simulink model "motor_1"  (R2023a)
settings: Solver=ode15s  StartTime=0.0  StopTime=sim_end_time  MaxStep=.0001  RelTol=1e-3
values from neighbouring files (symbols this model uses):
  alpha_cu = 3.9 *10^-3    (= 0.0039)    [BLDC_Motor_params_03.m]    (also in DC_Motor_params_01.m; DC_Motor_params_02.m; DC_Motor_params_04.m; DC_Motor_params_05.m)
  b_m1 = .01    (= 0.01)    [DC_Motor_params_01.m]
  C_t1 = 19.57    [DC_Motor_params_01.m]
  ENABLE_SATURATIONS = 1    [run_flags.m]
  J_eq1 = J_1 + 1/8 * m_1 * d_1^2 / r_1^2    [DC_Motor_params_01.m]
  K_d1 = 0.022261    [PID_tuning.m]
  k_e1 = 0.25    [DC_Motor_params_01.m]
  K_i1 = 0    [PID_tuning.m]
  K_p1 = 6.6674    [PID_tuning.m]
  k_t1 = 0.25    [DC_Motor_params_01.m]
  L_a1 = 7.5*10^-3    (= 0.0075)    [DC_Motor_params_01.m]
  r_1 = 25    [DC_Motor_params_01.m]
  r_a1_20 = 0.5    [DC_Motor_params_01.m]
  res_term_1 = 9.58    [DC_Motor_params_01.m]
  T_s0_1 = 20    [use_machine_1.m]    (also in use_solo_motor_1.m)
  theta_m0_1 = 0    [use_machine_1.m]    (also in use_solo_motor_1.m)
  voltage_1 = 12    [DC_Motor_params_01.m]
settings Model: Creator=Usuario  LastModifiedBy=Usuario

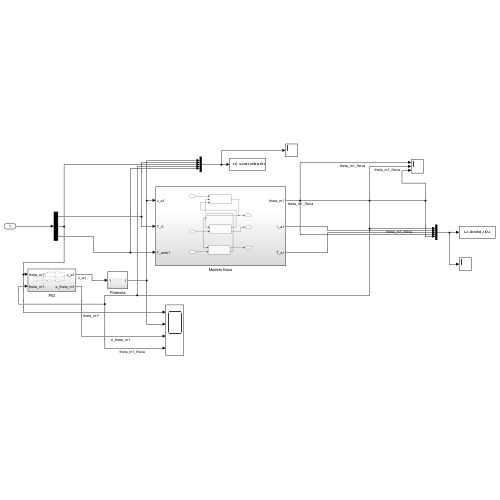
[thumbnail: Simulink's stored preview of the top-level diagram]
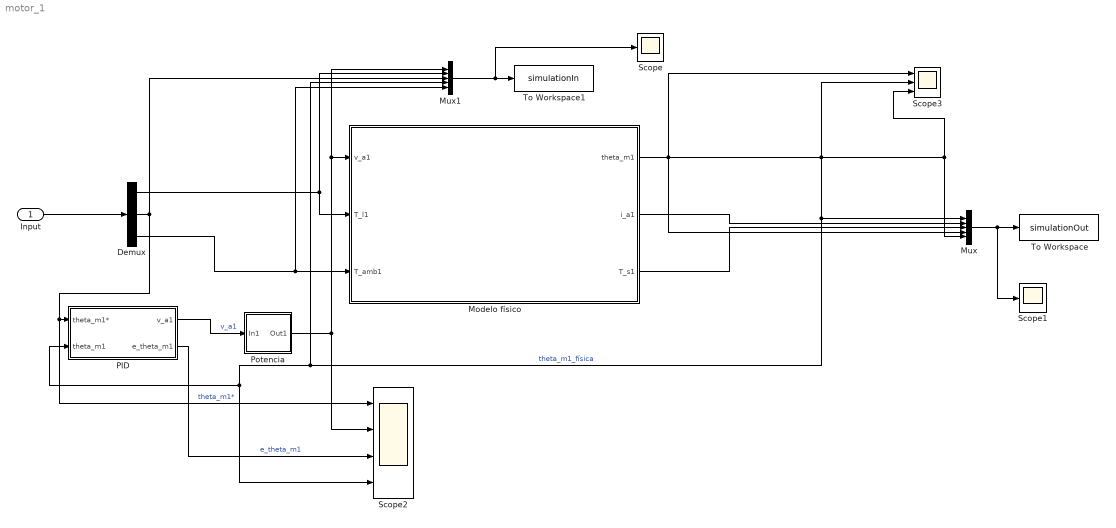
== system motor_1 ==
  Input : Inport
  Demux : Demux  Outputs=3
  Modelo físico : Subsystem
  Mux : Mux  Inputs=5
  Mux1 : Mux  Inputs=5
  PID : Subsystem
  Potencia : Subsystem
  Scope : Scope
  Scope1 : Scope
  Scope2 : Scope  NumInputPorts=4
  Scope3 : Scope  NumInputPorts=3
  To Workspace : ToWorkspace  VariableName=simulationOut  SaveFormat=Timeseries  SampleTime=-1
  To Workspace1 : ToWorkspace  VariableName=simulationIn  SaveFormat=Timeseries  SampleTime=-1
  wires:
  Demux/2 -> PID/1(theta_m1*), Scope2/1, Mux1/3  "theta_m1*"
  Mux1/1 -> Scope/1, To Workspace1/1
  Demux/1 -> Modelo físico/2(T_l1), Mux1/2
  Demux/3 -> Mux1/5, Modelo físico/3(T_amb1)
  Modelo físico/2(i_a1) -> Mux/2
  Mux/1 -> Scope1/1, To Workspace/1
  PID/1(v_a1) -> Potencia/1(In1)  "v_a1"
  PID/2(e_theta_m1) -> Scope2/3  "e_theta_m1"
  Modelo físico/3(T_s1) -> Mux/3
  Modelo físico/1(theta_m1) -> Mux/5, Scope3/3, Scope3/2, Scope2/4, PID/2(theta_m1), Mux1/4, Mux/1, Scope3/1, Mux/4  "theta_m1_física"
  Input/1 -> Demux/1
  Potencia/1(Out1) -> Modelo físico/1(v_a1), Mux1/1, Scope2/2

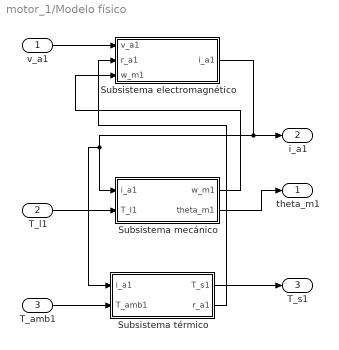
== system motor_1/Modelo físico ==
  v_a1 : Inport
  T_l1 : Inport  Port=2
  T_amb1 : Inport  Port=3
  Subsistema electromagnético : Subsystem
  Subsistema mecánico : Subsystem
  Subsistema térmico : Subsystem
  theta_m1 : Outport
  i_a1 : Outport  Port=2
  T_s1 : Outport  Port=3
  wires:
  Subsistema electromagnético/1(i_a1) -> Subsistema térmico/1(i_a1), Subsistema mecánico/1(i_a1), i_a1/1
  v_a1/1 -> Subsistema electromagnético/1(v_a1)
  T_l1/1 -> Subsistema mecánico/2(T_l1)
  T_amb1/1 -> Subsistema térmico/2(T_amb1)
  Subsistema térmico/1(T_s1) -> T_s1/1
  Subsistema térmico/2(r_a1) -> Subsistema electromagnético/2(r_a1)
  Subsistema mecánico/1(w_m1) -> Subsistema electromagnético/3(w_m1)
  Subsistema mecánico/2(theta_m1) -> theta_m1/1

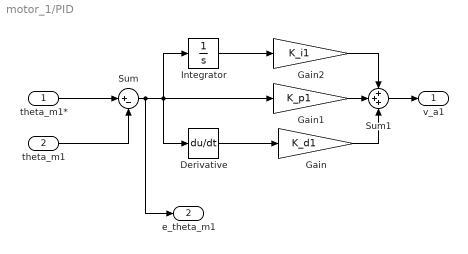
== system motor_1/PID ==
  theta_m1* : Inport
  theta_m1 : Inport  Port=2
  Derivative : Derivative
  Gain : Gain  Gain=K_d1
  Gain1 : Gain  Gain=K_p1
  Gain2 : Gain  Gain=K_i1
  Integrator : Integrator
  Sum : Sum  Inputs=|+-
  Sum1 : Sum  Inputs=+++
  v_a1 : Outport
  e_theta_m1 : Outport  Port=2
  wires:
  theta_m1*/1 -> Sum/1
  theta_m1/1 -> Sum/2
  Sum/1 -> e_theta_m1/1, Integrator/1, Gain1/1, Derivative/1
  Integrator/1 -> Gain2/1
  Derivative/1 -> Gain/1
  Gain1/1 -> Sum1/2
  Gain2/1 -> Sum1/1
  Sum1/1 -> v_a1/1
  Gain/1 -> Sum1/3

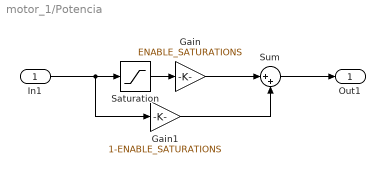
== system motor_1/Potencia ==
  In1 : Inport
  Gain : Gain  Gain=ENABLE_SATURATIONS
  Gain1 : Gain  Gain=1-ENABLE_SATURATIONS
  Saturation : Saturate  UpperLimit=+voltage_1  LowerLimit=-voltage_1
  Sum : Sum  Inputs=|++
  Out1 : Outport
  wires:
  In1/1 -> Gain1/1, Saturation/1
  Saturation/1 -> Gain/1
  Gain/1 -> Sum/1
  Sum/1 -> Out1/1
  Gain1/1 -> Sum/2

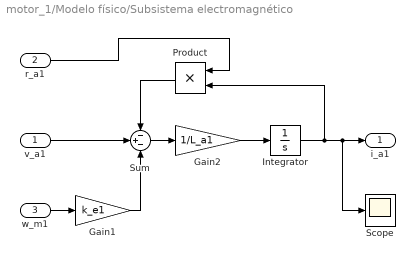
== system motor_1/Modelo físico/Subsistema electromagnético ==
  v_a1 : Inport
  r_a1 : Inport  Port=2
  w_m1 : Inport  Port=3
  Gain1 : Gain  Gain=k_e1
  Gain2 : Gain  Gain=1/L_a1
  Integrator : Integrator
  Product : Product
  Scope : Scope
  Sum : Sum  Inputs=-+-
  i_a1 : Outport
  wires:
  v_a1/1 -> Sum/2
  Integrator/1 -> Product/2, Scope/1, i_a1/1
  Product/1 -> Sum/1
  w_m1/1 -> Gain1/1
  Gain1/1 -> Sum/3
  Sum/1 -> Gain2/1
  Gain2/1 -> Integrator/1
  r_a1/1 -> Product/1

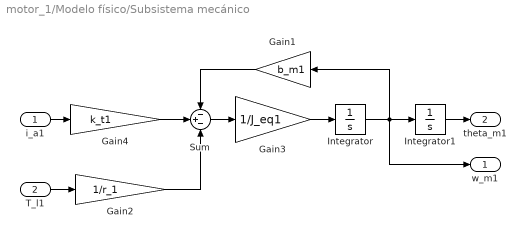
== system motor_1/Modelo físico/Subsistema mecánico ==
  i_a1 : Inport
  T_l1 : Inport  Port=2
  Gain1 : Gain  Gain=b_m1
  Gain2 : Gain  Gain=1/r_1
  Gain3 : Gain  Gain=1/J_eq1
  Gain4 : Gain  Gain=k_t1
  Integrator : Integrator
  Integrator1 : Integrator  InitialCondition=theta_m0_1
  Sum : Sum  Inputs=-+-
  w_m1 : Outport
  theta_m1 : Outport  Port=2
  wires:
  i_a1/1 -> Gain4/1
  Integrator/1 -> w_m1/1, Gain1/1, Integrator1/1
  Gain1/1 -> Sum/1
  T_l1/1 -> Gain2/1
  Gain3/1 -> Integrator/1
  Sum/1 -> Gain3/1
  Integrator1/1 -> theta_m1/1
  Gain2/1 -> Sum/3
  Gain4/1 -> Sum/2

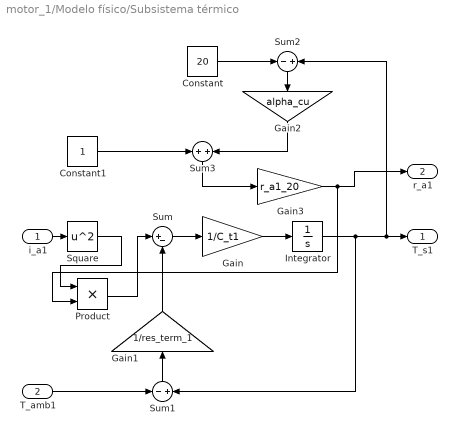
== system motor_1/Modelo físico/Subsistema térmico ==
  i_a1 : Inport
  T_amb1 : Inport  Port=2
  Constant : Constant  Value=20
  Constant1 : Constant
  Gain : Gain  Gain=1/C_t1
  Gain1 : Gain  Gain=1/res_term_1
  Gain2 : Gain  Gain=alpha_cu
  Gain3 : Gain  Gain=r_a1_20
  Integrator : Integrator  InitialCondition=T_s0_1
  Product : Product
  Square : Math  Operator=square
  Sum : Sum  Inputs=|+-
  Sum1 : Sum  Inputs=-|+
  Sum2 : Sum  Inputs=-|+
  Sum3 : Sum  Inputs=+|+
  T_s1 : Outport
  r_a1 : Outport  Port=2
  wires:
  i_a1/1 -> Square/1
  Sum3/1 -> Gain3/1
  Gain2/1 -> Sum3/2
  Square/1 -> Product/1
  Gain3/1 -> Product/2, r_a1/1
  Sum2/1 -> Gain2/1
  T_amb1/1 -> Sum1/1
  Constant1/1 -> Sum3/1
  Gain/1 -> Integrator/1
  Sum/1 -> Gain/1
  Integrator/1 -> Sum1/2, Sum2/2, T_s1/1
  Constant/1 -> Sum2/1
  Sum1/1 -> Gain1/1
  Gain1/1 -> Sum/2
  Product/1 -> Sum/1
